simulink model "sampleModel229"  (R2021b)
settings: Solver=VariableStepAuto  StartTime=0.0  StopTime=10.0  RelTol=1e-3
undefined symbols (not defined in the file or in its folder): Newton, Raphson
libraries: simulink x5
settings Model: Creator=user  LastModifiedBy=user

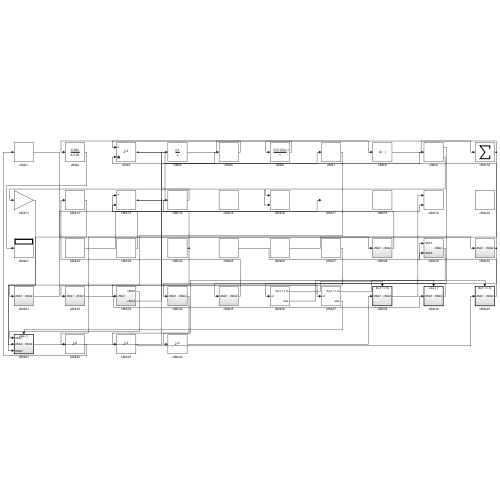
[thumbnail: Simulink's stored preview of the top-level diagram]
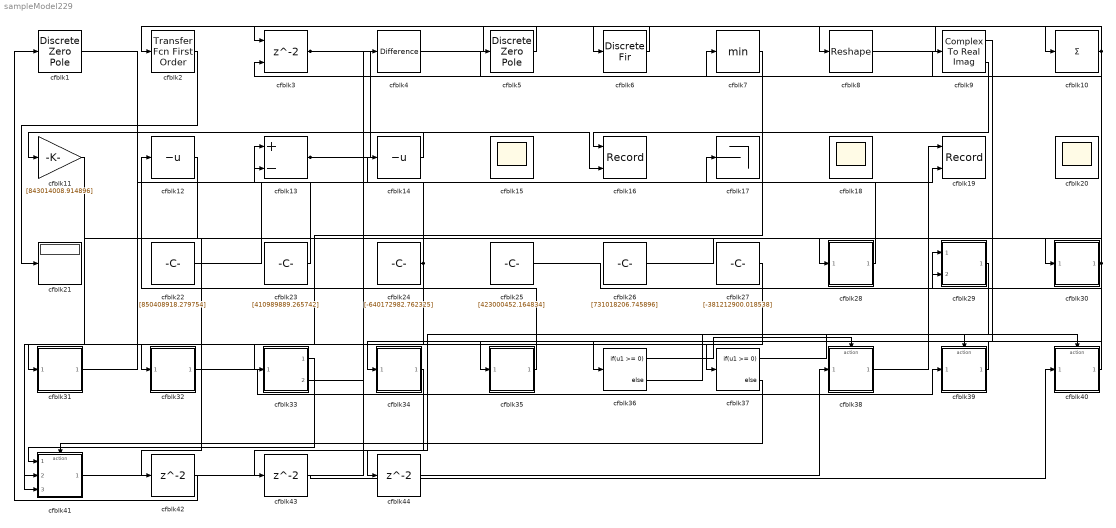
== system sampleModel229 ==
  cfblk1 : DiscreteZeroPole  Poles=[0 0.5]  Gain=1
  cfblk10 : Sum  Inputs=+
  cfblk11 : Gain  Gain=[843014008.914896]
  cfblk12 : UnaryMinus
  cfblk13 : Sum  Inputs=+-
  cfblk14 : UnaryMinus
  cfblk15 : Scope
      settings: Floating=on
  cfblk16 : Record  FileSettingsInternal="{\"entries\":[{\"content\":{\"excelSettings\":{\"content\":{},\"type\":\"Streamout.ExcelSettings\"}},\"type\":\"Streamout.FileSettingStorage\",\"uuid\":\"cca10b2c-9729-4ca0-a785-db39cad9df5a\"}],\"packageUris\":[\"http://schema.mathworks.com/mf0/streamout_blocks/R2020a\"],\"version\":\"1.0\"}"  Layout=[1 1]  SignalsInternal="{\"entries\":[{\"content\":{\"signals\":[{\"content\":{\"blockPath\":[\"sampleModel229/cfblk16\"],\"channel\":[],\"dimensions\":[1],\"domain\":\"sampleModel229/cfblk16\",\"lineColor\":\"#a2142f\",\"plots\":[1],\"port\":1,\"sid\":[\"\"],\"signalID\":8953,\"signalName\":\"cfblk9:2\"},\"type\":\"RecordBlkView.Signal\",\"uuid\":\"820c6719-806d-41ff-95bb-78ca30542d26\"},{\"content\":{\"blockPath\":[\"sampleModel229/cfblk16\"],\"channel\":[],\"dimensions\":[1],\"domain\":\"sampleModel229/cfblk16\",\"lineColor\":\"#139fff\",\"plots\":[1],\"port\":2,\"sid\":[\"\"],\"signalID\":8957,\"signalName\":\"cfblk3\"},\"type\":\"RecordBlkView.Signal\",\"uuid\":\"6f3903cd-712e-4836-be9f-ff089b180a78\"}]},\"type\":\"RecordBlkView.InputSignals\",\"uuid\":\"11a44d97-eb19-4198-bf9b-9edce6b18752\"}],\"packageUris\":[\"http://schema.mathworks.com/mf0/streamout_blocks/R2020a\"],\"version\":\"1.0\"}"  VisualizationBindings="{\"xyplotplugin\":{\"info\":[{\"series\":[{\"bindingParametersList\":[{\"parameter\":\"X-Axis\",\"signalID\":8953,\"signalName\":\"cfblk9:2\"},{\"parameter\":\"Y-Axis\",\"signalID\":8957,\"signalName\":\"cfblk3\"}],\"seriesID\":25820}],\"subplotID\":1}]}}"  CompatibilityTag=XY
  cfblk17 : Terminator
  cfblk18 : Scope
      settings: Floating=on
  cfblk19 : Record  FileSettingsInternal="{\"entries\":[{\"content\":{\"excelSettings\":{\"content\":{},\"type\":\"Streamout.ExcelSettings\"}},\"type\":\"Streamout.FileSettingStorage\",\"uuid\":\"69774671-d197-4a5b-883d-2b0e15201338\"}],\"packageUris\":[\"http://schema.mathworks.com/mf0/streamout_blocks/R2020a\"],\"version\":\"1.0\"}"  Layout=[1 1]  SignalsInternal="{\"entries\":[{\"content\":{\"signals\":[{\"content\":{\"blockPath\":[\"sampleModel229/cfblk19\"],\"channel\":[],\"dimensions\":[1],\"domain\":\"sampleModel229/cfblk19\",\"lineColor\":\"#a2142f\",\"plots\":[1],\"port\":1,\"sid\":[\"\"],\"signalID\":8961,\"signalName\":\"cfblk38\"},\"type\":\"RecordBlkView.Signal\",\"uuid\":\"76b91beb-2131-4cc8-8d98-00c31025ee17\"},{\"content\":{\"blockPath\":[\"sampleModel229/cfblk19\"],\"channel\":[],\"dimensions\":[1],\"domain\":\"sampleModel229/cfblk19\",\"lineColor\":\"#139fff\",\"plots\":[1],\"port\":2,\"sid\":[\"\"],\"signalID\":8965,\"signalName\":\"cfblk31\"},\"type\":\"RecordBlkView.Signal\",\"uuid\":\"71a84667-c1f3-487f-a230-678d0d5cdb25\"}]},\"type\":\"RecordBlkView.InputSignals\",\"uuid\":\"9fe9645a-9b05-4e15-8eb5-bc80d818af14\"}],\"packageUris\":[\"http://schema.mathworks.com/mf0/streamout_blocks/R2020a\"],\"version\":\"1.0\"}"  VisualizationBindings="{\"xyplotplugin\":{\"info\":[{\"series\":[{\"bindingParametersList\":[{\"parameter\":\"X-Axis\",\"signalID\":8961,\"signalName\":\"cfblk38\"},{\"parameter\":\"Y-Axis\",\"signalID\":8965,\"signalName\":\"cfblk31\"}],\"seriesID\":19951}],\"subplotID\":1}]}}"  CompatibilityTag=XY
  cfblk2 : simulink/Discrete/Transfer Fcn First Order  PoleZ=0.95  ICPrevOutput=0.0  DoSatur=off
  cfblk20 : Scope
      settings: Floating=on
  cfblk21 : Display
  cfblk22 : Constant  Value=[850408918.279754]  SampleTime=1
  cfblk23 : Constant  Value=[410989889.265742]  SampleTime=1
  cfblk24 : Constant  Value=[-640172982.762325]  SampleTime=1
  cfblk25 : Constant  Value=[423000452.164834]  SampleTime=1
  cfblk26 : Constant  Value=[731018206.745896]  SampleTime=1
  cfblk27 : Constant  Value=[-381212900.018538]  SampleTime=1
  cfblk28 : Subsystem
  cfblk29 : Subsystem
  cfblk3 : Delay  ShowEnablePort=on  SampleTime=1
      settings: InputPortMap=u0,e6
  cfblk30 : Subsystem
  cfblk31 : Subsystem
  cfblk32 : Subsystem
  cfblk33 : Subsystem
  cfblk34 : Subsystem
  cfblk35 : Subsystem
  cfblk36 : If  IfExpression=u1 >= 0  SampleTime=1
  cfblk37 : If  IfExpression=u1 >= 0  SampleTime=1
  cfblk38 : Subsystem  TreatAsAtomicUnit=on
  cfblk39 : Subsystem  TreatAsAtomicUnit=on
  cfblk4 : simulink/Discrete/Difference  ICPrevInput=0.0  OutMin=[]  OutMax=[]  OutDataTypeStr=Inherit: Inherit via back propagation  OutDataType=fixdt(1, 16)  OutScaling=2^-10  DoSatur=off
  cfblk40 : Subsystem  TreatAsAtomicUnit=on
  cfblk41 : Subsystem  TreatAsAtomicUnit=on
  cfblk42 : Delay  SampleTime=1
  cfblk43 : Delay  SampleTime=1
  cfblk44 : Delay  SampleTime=1
  cfblk5 : DiscreteZeroPole  Poles=[0 0.5]  Gain=1
  cfblk6 : DiscreteFir  SampleTime=1
  cfblk7 : MinMax
  cfblk8 : Reshape
  cfblk9 : ComplexToRealImag
  wires:
  cfblk14/1 -> cfblk11/1
  cfblk5/1 -> cfblk2/1
  cfblk32/1(cfblk2) -> cfblk39/1(cfblk1)
  cfblk39/1(cfblk2) -> cfblk34/1(cfblk1)
  cfblk26/1 -> cfblk30/1(cfblk1)
  cfblk9/1 -> cfblk35/1(cfblk1)
  cfblk22/1 -> cfblk17/1
  cfblk7/1 -> cfblk32/1(cfblk1)
  cfblk35/1(cfblk2) -> cfblk12/1
  cfblk40/1(cfblk2) -> cfblk29/1(cfblk1)
  cfblk3/1 -> cfblk7/1, cfblk16/2
  cfblk38/1(cfblk2) -> cfblk19/1
  cfblk23/1 -> cfblk13/1
  cfblk8/1 -> cfblk10/1
  cfblk4/1 -> cfblk8/1
  cfblk30/1(cfblk2) -> cfblk36/1, cfblk3/2
  cfblk2/1 -> cfblk21/1
  cfblk33/1(cfblk2) -> cfblk41/1(cfblk1)
  cfblk24/1 -> cfblk13/2, cfblk41/3(cfblk5)
  cfblk1/1 -> cfblk28/1(cfblk1)
  cfblk27/1 -> cfblk33/1(cfblk1)
  cfblk25/1 -> cfblk29/2(cfblk3)
  cfblk41/1(cfblk2) -> cfblk4/1
  cfblk12/1 -> cfblk31/1(cfblk1)
  cfblk10/1 -> cfblk6/1, cfblk42/1
  cfblk6/1 -> cfblk3/1
  cfblk33/2(cfblk4) -> cfblk9/1
  cfblk11/1 -> cfblk41/2(cfblk4)
  cfblk13/1 -> cfblk5/1, cfblk37/1
  cfblk31/1(cfblk2) -> cfblk19/2
  cfblk9/2 -> cfblk16/1
  cfblk28/1(cfblk2) -> cfblk14/1
  cfblk36/1 -> cfblk38/Action
  cfblk36/2 -> cfblk39/Action
  cfblk37/1 -> cfblk40/Action
  cfblk37/2 -> cfblk41/Action
  cfblk42/1 -> cfblk1/1
  cfblk34/1(cfblk2) -> cfblk43/1
  cfblk43/1 -> cfblk40/1(cfblk1)
  cfblk29/1(cfblk2) -> cfblk44/1
  cfblk44/1 -> cfblk38/1(cfblk1)

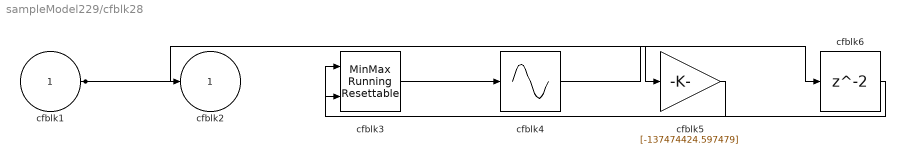
== system sampleModel229/cfblk28 ==
  cfblk1 : Inport
  cfblk3 : simulink/Math Operations/MinMax Running Resettable  Function=min  vinit=0.0
  cfblk4 : Sin  TimeSource=Use external signal  SampleTime=0
  cfblk5 : Gain  Gain=[-137474424.597479]
  cfblk6 : Delay  SampleTime=1
  cfblk2 : Outport
  wires:
  cfblk1/1 -> cfblk5/1, cfblk2/1
  cfblk5/1 -> cfblk3/1
  cfblk3/1 -> cfblk4/1
  cfblk4/1 -> cfblk6/1
  cfblk6/1 -> cfblk3/2

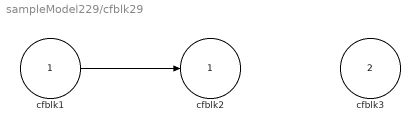
== system sampleModel229/cfblk29 ==
  cfblk1 : Inport
  cfblk3 : Inport  Port=2
  cfblk2 : Outport
  wires:
  cfblk1/1 -> cfblk2/1

== system sampleModel229/cfblk30 ==
  cfblk1 : Inport
  cfblk3 : Sum  Inputs=|++
  cfblk2 : Outport
  wires:
  cfblk1/1 -> cfblk3/1, cfblk3/2
  cfblk3/1 -> cfblk2/1

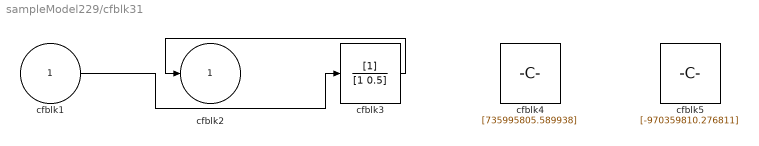
== system sampleModel229/cfblk31 ==
  cfblk1 : Inport
  cfblk3 : DiscreteFilter  SampleTime=1
  cfblk4 : Constant  Value=[735995805.589938]  SampleTime=1
  cfblk5 : Constant  Value=[-970359810.276811]  SampleTime=1
  cfblk2 : Outport
  wires:
  cfblk3/1 -> cfblk2/1
  cfblk1/1 -> cfblk3/1

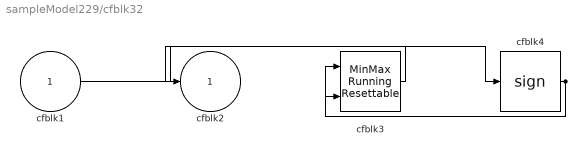
== system sampleModel229/cfblk32 ==
  cfblk1 : Inport
  cfblk3 : simulink/Math Operations/MinMax Running Resettable  Function=min  vinit=0.0
  cfblk4 : Signum
  cfblk2 : Outport
  wires:
  cfblk1/1 -> cfblk4/1
  cfblk4/1 -> cfblk3/1, cfblk3/2
  cfblk3/1 -> cfblk2/1

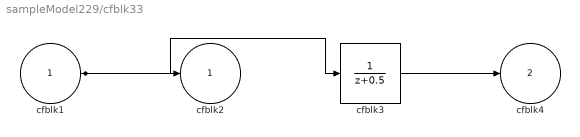
== system sampleModel229/cfblk33 ==
  cfblk1 : Inport
  cfblk3 : DiscreteTransferFcn  SampleTime=1
  cfblk2 : Outport
  cfblk4 : Outport  Port=2
  wires:
  cfblk3/1 -> cfblk4/1
  cfblk1/1 -> cfblk3/1, cfblk2/1

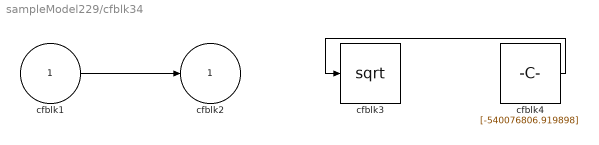
== system sampleModel229/cfblk34 ==
  cfblk1 : Inport
  cfblk3 : Sqrt  SaturateOnIntegerOverflow=on
  cfblk4 : Constant  Value=[-540076806.919898]  SampleTime=1
  cfblk2 : Outport
  wires:
  cfblk4/1 -> cfblk3/1
  cfblk1/1 -> cfblk2/1

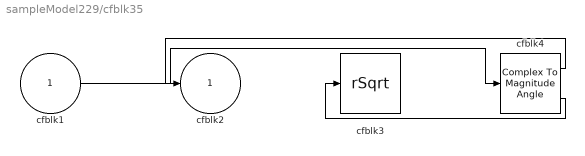
== system sampleModel229/cfblk35 ==
  cfblk1 : Inport
  cfblk3 : Sqrt  Operator=rSqrt  AlgorithmType=Newton-Raphson  SaturateOnIntegerOverflow=on
  cfblk4 : ComplexToMagnitudeAngle
  cfblk2 : Outport
  wires:
  cfblk1/1 -> cfblk4/1
  cfblk4/1 -> cfblk2/1
  cfblk4/2 -> cfblk3/1

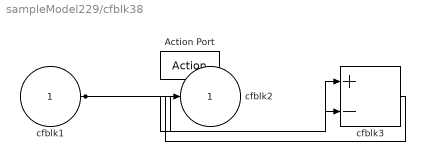
== system sampleModel229/cfblk38 ==
  cfblk1 : Inport
  Action Port : ActionPort  ActionPortLabel=if(u1 >= 0)
  cfblk3 : Sum  Inputs=+-
  cfblk2 : Outport
  wires:
  cfblk1/1 -> cfblk3/1, cfblk3/2
  cfblk3/1 -> cfblk2/1

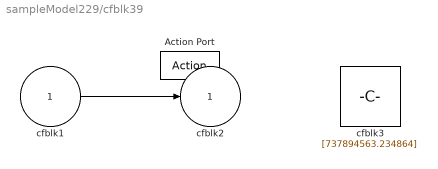
== system sampleModel229/cfblk39 ==
  cfblk1 : Inport
  Action Port : ActionPort  ActionPortLabel=else
  cfblk3 : Constant  Value=[737894563.234864]  SampleTime=1
  cfblk2 : Outport
  wires:
  cfblk1/1 -> cfblk2/1

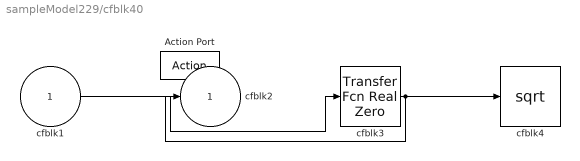
== system sampleModel229/cfblk40 ==
  cfblk1 : Inport
  Action Port : ActionPort  ActionPortLabel=if(u1 >= 0)
  cfblk3 : simulink/Discrete/Transfer Fcn Real Zero  ZeroZ=0.75  ICPrevInput=0.0  DoSatur=off
      settings: SourceProductBaseCode=SL
  cfblk4 : Sqrt  SaturateOnIntegerOverflow=on
  cfblk2 : Outport
  wires:
  cfblk1/1 -> cfblk3/1
  cfblk3/1 -> cfblk2/1, cfblk4/1

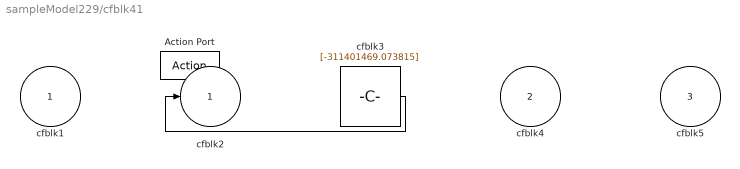
== system sampleModel229/cfblk41 ==
  cfblk1 : Inport
  cfblk4 : Inport  Port=2
  cfblk5 : Inport  Port=3
  Action Port : ActionPort  ActionPortLabel=else
  cfblk3 : Constant  Value=[-311401469.073815]  SampleTime=1
  cfblk2 : Outport
  wires:
  cfblk3/1 -> cfblk2/1
